simulink model "FutureGridSLs"  (R2024a)
settings: Solver=VariableStepAuto  StartTime=0.0  StopTime=600  FixedStep=1e-3  RelTol=1e-3
values from neighbouring files (symbols this model uses):
  AGG_SOL_R = inf    [FUtureGridSL.m]
  AGG_SOL_S_nom = 980e6    (= 980000000)    [FUtureGridSL.m]
  AGG_SOL_T_INV = 0.02    [FUtureGridSL.m]
  AMB_T_INV = 0.05    [FUtureGridSL.m]
  AMB_Unit_S_nom = 3e6    (= 3000000)    [FUtureGridSL.m]
  BAR_R = 0.04    [FUtureGridSL.m]
  BAR_T_ACT = 0.1    [FUtureGridSL.m]
  BAR_Unit_S_nom = 15e6    (= 15000000)    [FUtureGridSL.m]
  BRO_R_P = 0.05    [FUtureGridSL.m]    (also in Sri_Lanka_FINAL.m)
  BRO_R_T = 0.38    [FUtureGridSL.m]    (also in Sri_Lanka_FINAL.m)
  BRO_T_G = 0.2    [FUtureGridSL.m]    (also in Sri_Lanka_FINAL.m)
  BRO_T_R = 5.0    (= 5)    [FUtureGridSL.m]    (also in Sri_Lanka_FINAL.m)
  BRO_T_W = 1.0    (= 1)    [FUtureGridSL.m]    (also in Sri_Lanka_FINAL.m)
  BRO_Unit_S_nom = 17.5e6    (= 17500000)    [FUtureGridSL.m]    (also in Sri_Lanka_FINAL.m)
  BWT_R_P = 0.05    [FUtureGridSL.m]    (also in Sri_Lanka.m; Sri_Lanka_FINAL.m)
  BWT_R_T = 0.38    [FUtureGridSL.m]    (also in Sri_Lanka.m; Sri_Lanka_FINAL.m)
  BWT_T_R = 5.0    (= 5)    [FUtureGridSL.m]    (also in Sri_Lanka.m; Sri_Lanka_FINAL.m)
  BWT_T_W = 1.5    [FUtureGridSL.m]    (also in Sri_Lanka.m; Sri_Lanka_FINAL.m)
  BWT_Unit_S_nom = 40e6    (= 40000000)    [FUtureGridSL.m]    (also in Sri_Lanka.m; Sri_Lanka_FINAL.m)
  CAN_R_P = 0.05    [FUtureGridSL.m]    (also in Sri_Lanka_FINAL.m)
  CAN_R_T = 0.38    [FUtureGridSL.m]    (also in Sri_Lanka_FINAL.m)
  CAN_T_G = 0.2    [FUtureGridSL.m]    (also in Sri_Lanka_FINAL.m)
  CAN_T_R = 5.0    (= 5)    [FUtureGridSL.m]    (also in Sri_Lanka_FINAL.m)
  CAN_T_W = 1.0    (= 1)    [FUtureGridSL.m]    (also in Sri_Lanka_FINAL.m)
  CAN_Unit_S_nom = 30e6    (= 30000000)    [FUtureGridSL.m]    (also in Sri_Lanka_FINAL.m)
  D_T = 1500e6/S_base_sys    (= 1.5)    [FUtureGridSL.m]    (also in Sri_Lanka.m; Sri_Lanka_FINAL.m)
  f_base = 50    [FUtureGridSL.m]    (also in Sri_Lanka.m; Sri_Lanka_FINAL.m)
  H_eq = sum(Plant_H .* Plant_S_nom .* Plant_Status) / S_base_sys    [FUtureGridSL.m]    (also in Sri_Lanka.m = sum(Plant_H .* Plant_S_nom) / S_base_sys; Sri_Lanka_FINAL.m = sum(Plant_H .* Plant_S_nom) / S_base_sys)
  HBT_S_nom = 1.2e6    (= 1200000)    [FUtureGridSL.m]
  HBT_T_INV = 0.02    [FUtureGridSL.m]
  KEL_CC_F_GT = 0.67    [FUtureGridSL.m]    (also in Sri_Lanka.m; Sri_Lanka_FINAL.m)
  KEL_CC_F_ST = 0.33    [FUtureGridSL.m]    (also in Sri_Lanka.m; Sri_Lanka_FINAL.m)
  KEL_CC_T_HRSG = 10.0    (= 10)    [FUtureGridSL.m]    (also in Sri_Lanka.m; Sri_Lanka_FINAL.m)
  KEL_R = 0.04    [FUtureGridSL.m]    (also in Sri_Lanka.m; Sri_Lanka_FINAL.m)
  KEL_T_CH = 0.3    [FUtureGridSL.m]    (also in Sri_Lanka.m; Sri_Lanka_FINAL.m)
  KEL_UNIT1_S_nom = 20e6    (= 20000000)    [FUtureGridSL.m]    (also in Sri_Lanka.m; Sri_Lanka_FINAL.m)
  KEL_UNIT2_S_nom = 115e6    (= 115000000)    [FUtureGridSL.m]    (also in Sri_Lanka.m; Sri_Lanka_FINAL.m)
  KEL_UNIT3_S_nom = 165e6    (= 165000000)    [FUtureGridSL.m]    (also in Sri_Lanka.m; Sri_Lanka_FINAL.m)
  KOT_R_P = 0.05    [FUtureGridSL.m]
  KOT_R_T = 0.38    [FUtureGridSL.m]
  KOT_T_R = 5.0    (= 5)    [FUtureGridSL.m]
  KOT_T_W = 1.1    [FUtureGridSL.m]
  KOT_Unit_S_nom = 67e6    (= 67000000)    [FUtureGridSL.m]
  KUK_R_P = 0.05    [FUtureGridSL.m]    (also in Sri_Lanka_FINAL.m)
  KUK_R_T = 0.38    [FUtureGridSL.m]    (also in Sri_Lanka_FINAL.m)
  KUK_T_R = 5.0    (= 5)    [FUtureGridSL.m]    (also in Sri_Lanka_FINAL.m)
  KUK_T_W = 0.8    [FUtureGridSL.m]    (also in Sri_Lanka_FINAL.m)
  KUK_Unit_S_nom = 40e6    (= 40000000)    [FUtureGridSL.m]    (also in Sri_Lanka_FINAL.m)
  LAK_R = 0.04    [FUtureGridSL.m]    (also in Sri_Lanka.m; Sri_Lanka_FINAL.m)
  LAK_S_nom = 300e6    (= 300000000)    [FUtureGridSL.m]    (also in Sri_Lanka.m; Sri_Lanka_FINAL.m)
  LAU_T_INV = 0.02    [FUtureGridSL.m]
  LAU_Unit_S_nom = 20e6    (= 20000000)    [FUtureGridSL.m]
  Load_pu = 2388.8 / 1000    (= 2.3888)    [FUtureGridSL.m]
  MAD_T_INV = 0.02    [FUtureGridSL.m]
  MAD_Unit_S_nom = 100e6    (= 100000000)    [FUtureGridSL.m]
  MADK_Unit_S_nom = 12e6    (= 12000000)    [FUtureGridSL.m]
  MADU_T_INV = 0.05    [FUtureGridSL.m]
  MAM1_T_INV = 0.05    [FUtureGridSL.m]
  MAM1_Unit_S_nom = 10e6    (= 10000000)    [FUtureGridSL.m]
  MAM2_T_INV = 0.05    [FUtureGridSL.m]
  MAM2_Unit_S_nom = 10e6    (= 10000000)    [FUtureGridSL.m]
  MAM3_T_INV = 0.05    [FUtureGridSL.m]
  MAM3_Unit_S_nom = 10e6    (= 10000000)    [FUtureGridSL.m]
  MAN_T_INV = 0.05    [FUtureGridSL.m]    (also in Sri_Lanka_FINAL.m)
  MAN_Unit_S_nom = 100e6    (= 100000000)    [FUtureGridSL.m]    (also in Sri_Lanka_FINAL.m)
  NAL_T_INV = 0.05    [FUtureGridSL.m]
  NAL_Unit_S_nom = 4.8e6    (= 4800000)    [FUtureGridSL.m]
  NIR_T_INV = 0.05    [FUtureGridSL.m]
  NIR_Unit_S_nom = 10.5e6    (= 10500000)    [FUtureGridSL.m]
  NLX_R_P = 0.05    [FUtureGridSL.m]    (also in Sri_Lanka_FINAL.m)
  NLX_R_T = 0.40    (= 0.4)    [FUtureGridSL.m]    (also in Sri_Lanka_FINAL.m)
  NLX_T_G = 0.2    [FUtureGridSL.m]    (also in Sri_Lanka_FINAL.m)
  NLX_T_R = 5.0    (= 5)    [FUtureGridSL.m]    (also in Sri_Lanka_FINAL.m)
  NLX_T_W = 1.2    [FUtureGridSL.m]    (also in Sri_Lanka_FINAL.m)
  NLX_Unit_S_nom = 50e6    (= 50000000)    [FUtureGridSL.m]    (also in Sri_Lanka_FINAL.m)
  OLX_R_P = 0.05    [FUtureGridSL.m]    (also in Sri_Lanka_FINAL.m)
  OLX_R_T = 0.38    [FUtureGridSL.m]    (also in Sri_Lanka_FINAL.m)
  OLX_T_G = 0.2    [FUtureGridSL.m]    (also in Sri_Lanka_FINAL.m)
  OLX_T_R = 5.0    (= 5)    [FUtureGridSL.m]    (also in Sri_Lanka_FINAL.m)
  OLX_T_W = 1.0    (= 1)    [FUtureGridSL.m]    (also in Sri_Lanka_FINAL.m)
  OLX_Unit_S_nom_1 = 12.5e6    (= 12500000)    [FUtureGridSL.m]    (also in Sri_Lanka_FINAL.m)
  OLX_Unit_S_nom_2 = 8.33e6    (= 8330000)    [FUtureGridSL.m]    (also in Sri_Lanka_FINAL.m)
  POL_R_P = 0.05    [FUtureGridSL.m]    (also in Sri_Lanka_FINAL.m)
  POL_R_T = 0.40    (= 0.4)    [FUtureGridSL.m]    (also in Sri_Lanka_FINAL.m)
  POL_T_G = 0.2    [FUtureGridSL.m]    (also in Sri_Lanka_FINAL.m)
  POL_T_R = 5.0    (= 5)    [FUtureGridSL.m]    (also in Sri_Lanka_FINAL.m)
  POL_T_W = 1.4    [FUtureGridSL.m]    (also in Sri_Lanka_FINAL.m)
  POL_Unit_S_nom = 45e6    (= 45000000)    [FUtureGridSL.m]    (also in Sri_Lanka_FINAL.m)
  POLW_T_INV = 0.05    [FUtureGridSL.m]
  POLW_Unit_S_nom = 12e6    (= 12000000)    [FUtureGridSL.m]
  Pref_Set_AGG_SOL = (Load_pu * K_AGG_SOL)  * (S_base_sys / AGG_SOL_S_nom)    (= 0)    [FUtureGridSL.m]
  Pref_Set_AMB = (Load_pu * K_AMB) * (S_base_sys / AMB_Unit_S_nom)    (= 0)    [FUtureGridSL.m]
  Pref_Set_BAR = (Load_pu * K_BAR) * (S_base_sys / (4 * BAR_Unit_S_nom))    (= 3.98133333333)    [FUtureGridSL.m]
  Pref_Set_BRO = (Load_pu * K_BRO) * (S_base_sys / (2 * BRO_Unit_S_nom))    (= 0)    [FUtureGridSL.m]
  Pref_Set_BWT = (Load_pu * K_BWT) * (S_base_sys / (1 * BWT_Unit_S_nom))    (= 0)    [FUtureGridSL.m]
  Pref_Set_CAN = (Load_pu * K_CAN) * (S_base_sys / (2 * CAN_Unit_S_nom))    (= 0)    [FUtureGridSL.m]
  Pref_Set_HBT = (Load_pu * K_HBT)  * (S_base_sys / HBT_S_nom)    (= 0)    [FUtureGridSL.m]
  Pref_Set_KEL1 = (Load_pu * K_KEL1)  * (S_base_sys / (4*KEL_UNIT1_S_nom))    (= 0)    [FUtureGridSL.m]
  Pref_Set_KEL2 = (Load_pu * K_KEL2)  * (S_base_sys / (KEL_UNIT2_S_nom ))    (= 0)    [FUtureGridSL.m]
  Pref_Set_KEL3 = (Load_pu * K_KEL3)  * (S_base_sys / (KEL_UNIT3_S_nom))    (= 0)    [FUtureGridSL.m]
  Pref_Set_KOT = (Load_pu * K_KOT)  * (S_base_sys / (3 * KOT_Unit_S_nom))    (= 0.986419900498)    [FUtureGridSL.m]
  Pref_Set_KUK = (Load_pu * K_KUK) * (S_base_sys / (2 * KUK_Unit_S_nom))    (= 0)    [FUtureGridSL.m]
  Pref_Set_LAK = (Load_pu * K_LAK)  * (S_base_sys / (3 * LAK_S_nom))    (= 0.177302044444)    [FUtureGridSL.m]
  Pref_Set_LAU = (Load_pu * K_LAU)  * (S_base_sys / LAU_Unit_S_nom)    (= 1.1944)    [FUtureGridSL.m]
  Pref_Set_MAD = (Load_pu * K_MAD)  * (S_base_sys / MAD_Unit_S_nom)    (= 0.7333616)    [FUtureGridSL.m]
  Pref_Set_MADK = (Load_pu * K_MADK) * (S_base_sys / AMB_Unit_S_nom)    (= 0)    [FUtureGridSL.m]
  Pref_Set_MAM1 = (Load_pu * K_MAM1) * (S_base_sys / MAM1_Unit_S_nom)    (= 0)    [FUtureGridSL.m]
  Pref_Set_MAM2 = (Load_pu * K_MAM2) * (S_base_sys / MAM2_Unit_S_nom)    (= 0)    [FUtureGridSL.m]
  Pref_Set_MAM3 = (Load_pu * K_MAM3) * (S_base_sys / MAM3_Unit_S_nom)    (= 0)    [FUtureGridSL.m]
  Pref_Set_MAN = (Load_pu * K_MAN)  * (S_base_sys / MAN_Unit_S_nom)    (= 0.035832)    [FUtureGridSL.m]
  Pref_Set_NAL = (Load_pu * K_NAL) * (S_base_sys / NAL_Unit_S_nom)    (= 0)    [FUtureGridSL.m]
  Pref_Set_NIR = (Load_pu * K_NIR) * (S_base_sys / NIR_Unit_S_nom)    (= 0)    [FUtureGridSL.m]
  Pref_Set_NLX = (Load_pu * K_NLX)  * (S_base_sys / (2 * NLX_Unit_S_nom))    (= 0)    [FUtureGridSL.m]
  Pref_Set_OLX1 = (Load_pu * K_OLX1) * (S_base_sys / (2 * OLX_Unit_S_nom_1))    (= 0)    [FUtureGridSL.m]
  Pref_Set_OLX2 = (Load_pu * K_OLX2) * (S_base_sys / (3 * OLX_Unit_S_nom_2))    (= 0)    [FUtureGridSL.m]
  Pref_Set_POL = (Load_pu * K_POL) * (S_base_sys / (2 * POL_Unit_S_nom))    (= 0)    [FUtureGridSL.m]
  Pref_Set_POLW = (Load_pu * K_POLW) * (S_base_sys / POLW_Unit_S_nom)    (= 0)    [FUtureGridSL.m]
  Pref_Set_PWD = (Load_pu * K_PWD) * (S_base_sys / PWD_Unit_S_nom)    (= 0)    [FUtureGridSL.m]
  Pref_Set_RAN = (Load_pu * K_RAN) * (S_base_sys / (2 * RAN_Unit_S_nom))    (= 9.47936507937)    [FUtureGridSL.m]
  Pref_Set_RTB = (Load_pu * K_RTB) * (S_base_sys / (2 * RTB_Unit_S_nom))    (= 0)    [FUtureGridSL.m]
  ... (+116 more)
(part 1 of 2)
settings Model: Creator=munas  LastModifiedBy=munas

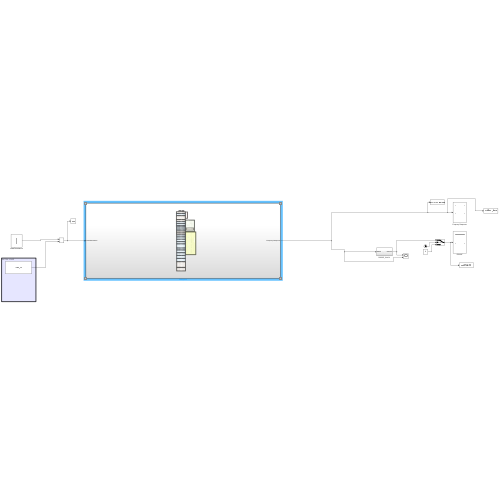
[thumbnail: Simulink's stored preview of the top-level diagram]
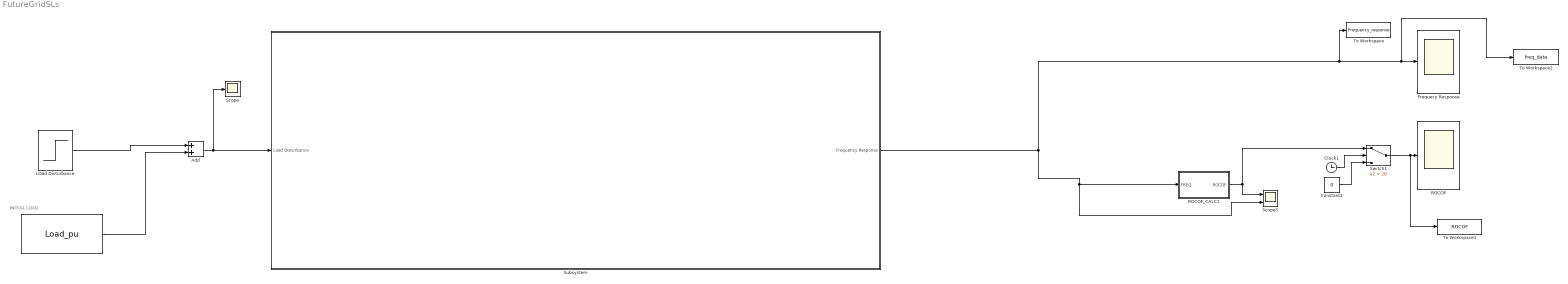
== system FutureGridSLs ==
  note: INITIAL LOAD
  "  " : Constant  Value=Load_pu
  Add : Sum
  Clock1 : Clock
  Constant2 : Constant  Value=0
  Frequecy Response : Scope
  LOad Disturbance : Step  Time=t_dist +200  After=150e6/S_base_sys  SampleTime=0
  ROCOF : Scope
  ROCOF_CALC1 : Subsystem
  Scope : Scope
  Scope5 : Scope  NumInputPorts=2
  Subsystem : Subsystem
  Switch1 : Switch  Criteria=u2 > Threshold  Threshold=20  SaturateOnIntegerOverflow=off  InputSameDT=off
  To Workspace : ToWorkspace  VariableName=Frequency_response  SaveFormat=Timeseries  SampleTime=-1
  To Workspace1 : ToWorkspace  VariableName=ROCOF  SaveFormat=Timeseries  SampleTime=-1
  To Workspace2 : ToWorkspace  VariableName=freq_data  SaveFormat=Timeseries  SampleTime=-1
  wires:
  Subsystem/1(Frequency Response) -> Scope5/2, ROCOF_CALC1/1(FREQ), To Workspace/1, To Workspace2/1, Frequecy Response/1
  Constant2/1 -> Switch1/3
  Switch1/1 -> To Workspace1/1, ROCOF/1
  Clock1/1 -> Switch1/2
  ROCOF_CALC1/1(ROCOF) -> Switch1/1, Scope5/1
  "  "/1 -> Add/2
  Add/1 -> Scope/1, Subsystem/1(Load Disturbance)
  LOad Disturbance/1 -> Add/1

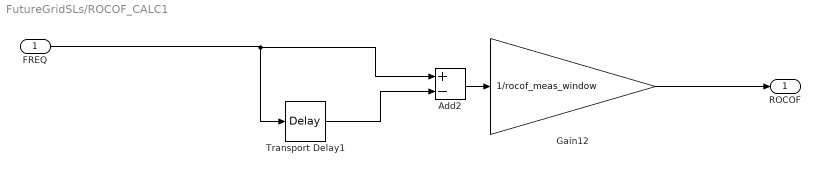
== system FutureGridSLs/ROCOF_CALC1 ==
  FREQ : Inport
  Add2 : Sum  Inputs=+-
  Gain12 : Gain  Gain=1/rocof_meas_window
  Transport Delay1 : TransportDelay  DelayTime=rocof_meas_window  InitialOutput=50
  ROCOF : Outport
  wires:
  Transport Delay1/1 -> Add2/2
  Gain12/1 -> ROCOF/1
  Add2/1 -> Gain12/1
  FREQ/1 -> Add2/1, Transport Delay1/1
